simulink model "gm_CornerDetection"  (R2019b)
settings: Solver=FixedStepDiscrete  StartTime=0.0  StopTime=Ts_240p*5  RelTol=1e-3
InitFcn:
  | Ts = 1e-3;
  | Ts_240p = 402*324*Ts;
  | Ts_480p = 525*800*Ts;
undefined symbols (not defined in the file or in its folder): fspecial, gray, Rec, SDTV
libraries: hdlsllib x8, visionhdlfilter x5, visionhdlio x2, simulink x1, visionhdlutilities x1, visionhdlconversions x1, dspvision x1
settings Model: ModifiedByFormat=The MathWorks Inc.  Creator=The MathWorks, Inc.  LastModifiedBy=The MathWorks Inc.
settings DataIOCC: LimitDataPoints=on  SaveFormat=Array  SaveOutput=off  SaveTime=off  ReturnWorkspaceOutputs=off
settings OptimizationCC: BlockReduction=off  ConditionallyExecuteInputs=off  DefaultParameterBehavior=Inlined  LifeSpan=inf
settings DebuggingCC: AlgebraicLoopMsg=error  SolverPrmCheckMsg=warning  InheritedTsInSrcMsg=none  SingleTaskRateTransMsg=error  ParameterPrecisionLossMsg=none  AllowSymbolicDim=off  SFUnexpectedBacktrackingDiag=warning  SFNoUnconditionalDefaultTransitionDiag=warning  SFExecutionAtInitializationDiag=none  IntegerSaturationMsg=none  ArithmeticOperatorsInVariantConditions=warning
settings HardwareCC: ProdBitPerPointer=32  ProdBitPerSizeT=32  ProdBitPerPtrDiffT=32  ProdLargestAtomicFloat=None  ProdIntDivRoundTo=Undefined  ProdEndianess=Unspecified  ProdWordSize=32  ProdHWDeviceType=ASIC/FPGA->ASIC/FPGA  ProdEqTarget=off
settings ModelReferenceCC: PropagateSignalLabelsOutOfModel=off
settings SFSimCC: SimUseLocalCustomCode=off  CustomCodeUndefinedFunction=UseInterfaceOnly
settings RTWCC: RTWUseLocalCustomCode=off
settings CodeAppCC: StateflowObjectComments=on
settings GRTTargetCC: TargetLangStandard=C89/C90 (ANSI)  GeneratePreprocessorConditionals=Disable all
settings ConfigComp: CovMetricSettings=dw  CovHtmlReporting=on  CovSaveCumulativeToWorkspaceVar=on  CovSaveSingleToWorkspaceVar=on  CovShowResultsExplorer=off  CovExternalEMLEnable=off  CovSFcnEnable=off

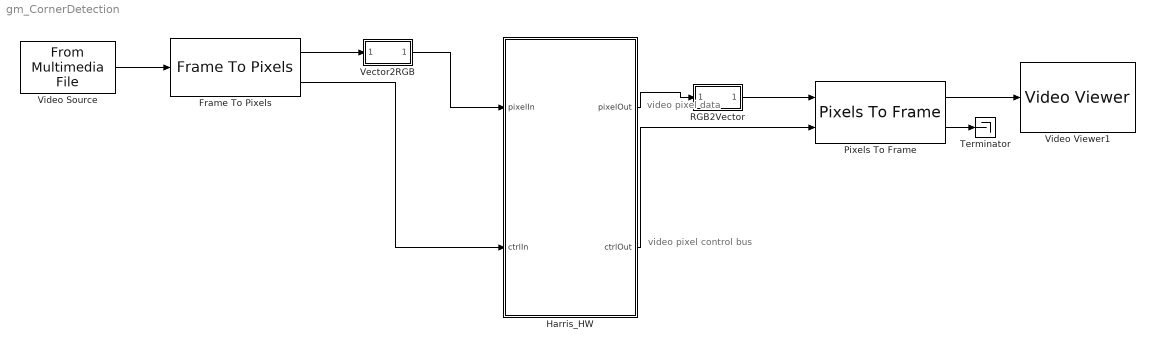
== system gm_CornerDetection ==
  note: video pixel control bus
  note: video pixel data
  Frame To Pixels : visionhdlio/Frame To Pixels  NumComponents=3  NumPixels=1  VideoFormat=480p  ActivePixelsPerLine=32  ActiveVideoLines=18  TotalPixelsPerLine=42  TotalVideoLines=28  StartingActiveLine=6  FrontPorch=5  SampleTime=0
      settings: SourceProductName=Vision HDL Toolbox  SourceProductBaseCode=VT
  Harris_HW : Subsystem  TreatAsAtomicUnit=on
  Pixels To Frame : visionhdlio/Pixels To Frame  NumComponents=3  NumPixels=1  VideoFormat=480p  ActivePixelsPerLine=32  ActiveVideoLines=18  TotalPixelsPerLine=42  TotalVideoLines=28
      settings: SourceProductName=Vision HDL Toolbox  SourceProductBaseCode=VT
  RGB2Vector : Subsystem
  Terminator : Terminator
  Vector2RGB : Subsystem
  Video Source : dspvision/From Multimedia File  inputFilename=D:\RnD\Current_Projects\Musawwir\Frameworks\HW\Musawwir_HW_Zedboard\Custom_IP_Cores\Matlab\Harris\test.jpg  readRange=[1 Inf]  loop=on  numPlays=inf  outputStreams=Video only  videoDataType=uint8  audioDataType=int16  inheritSampleTime=off  userDefinedSampleTime=Ts_480p  noAudioOutput=off  isIntensityVideo=off  fourcc=RGB  colorVideoFormat=One multidimensional signal  outputEOF=off  dataOrg=Column-major  audioFrameSize=1024  computeAudioFrameSize=off  outSamplingMode=Sample based
      settings: SourceProductName=Computer Vision Toolbox  SourceProductBaseCode=VP
  Video Viewer1 : VideoViewer  colormapValue=gray(256)  FigPos=[430.6 726 588 436]
  wires:
  Harris_HW/2(ctrlOut) -> Pixels To Frame/2
  Frame To Pixels/2 -> Harris_HW/2(ctrlIn)
  RGB2Vector/1(RGBVector) -> Pixels To Frame/1
  Frame To Pixels/1 -> Vector2RGB/1(RGBVector)
  Video Source/1 -> Frame To Pixels/1
  Harris_HW/1(pixelOut) -> RGB2Vector/1(RGB)
  Vector2RGB/1(RGB) -> Harris_HW/1(pixelIn)
  Pixels To Frame/1 -> Video Viewer1/1
  Pixels To Frame/2 -> Terminator/1

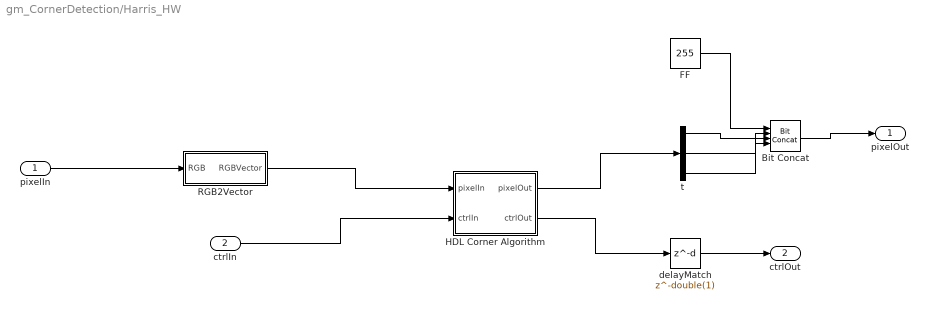
== system gm_CornerDetection/Harris_HW ==
  pixelIn : Inport  OutDataTypeStr=uint32  PortDimensions=1  SampleTime=0.001
  ctrlIn : Inport  Port=2  SampleTime=0.001
  Bit Concat : hdlsllib/Logic and Bit Operations/Bit Concat  numInputs=4
      settings: SourceProductName=Simulink
  FF : Constant  Value=255  OutDataTypeStr=uint8  SampleTime=-1
  HDL Corner Algorithm : Subsystem
  RGB2Vector : Subsystem
  delayMatch : Delay  DelayLength=double(1)  InitialCondition=0  SampleTime=0.001
  t : Demux  Outputs=3
  pixelOut : Outport  VectorParamsAs1DForOutWhenUnconnected=off
  ctrlOut : Outport  Port=2  VectorParamsAs1DForOutWhenUnconnected=off
  wires:
  pixelIn/1 -> RGB2Vector/1(RGB)
  ctrlIn/1 -> HDL Corner Algorithm/2(ctrlIn)
  Bit Concat/1 -> pixelOut/1
  FF/1 -> Bit Concat/1
  HDL Corner Algorithm/1(pixelOut) -> t/1
  delayMatch/1 -> ctrlOut/1
  RGB2Vector/1(RGBVector) -> HDL Corner Algorithm/1(pixelIn)
  t/1 -> Bit Concat/2
  t/2 -> Bit Concat/3
  t/3 -> Bit Concat/4
  HDL Corner Algorithm/2(ctrlOut) -> delayMatch/1

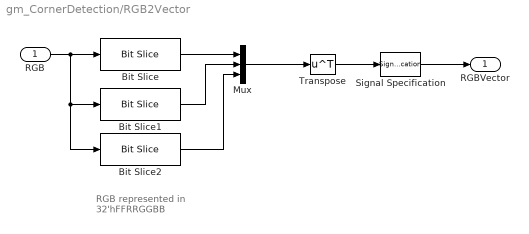
== system gm_CornerDetection/RGB2Vector ==
  note: RGB represented in
      | 32'hFFRRGGBB
  RGB : Inport
  Bit Slice : hdlsllib/Logic and Bit Operations/Bit Slice  lidx=23  ridx=16
  Bit Slice1 : hdlsllib/Logic and Bit Operations/Bit Slice  lidx=15  ridx=8
  Bit Slice2 : hdlsllib/Logic and Bit Operations/Bit Slice  lidx=7  ridx=0
  Mux : Mux  Inputs=3
  Signal Specification : SignalSpecification
  Transpose : Math  Operator=transpose  SaturateOnIntegerOverflow=on
  RGBVector : Outport  VectorParamsAs1DForOutWhenUnconnected=off
  wires:
  Signal Specification/1 -> RGBVector/1
  Transpose/1 -> Signal Specification/1
  RGB/1 -> Bit Slice/1, Bit Slice1/1, Bit Slice2/1
  Bit Slice1/1 -> Mux/2
  Bit Slice2/1 -> Mux/3
  Bit Slice/1 -> Mux/1
  Mux/1 -> Transpose/1

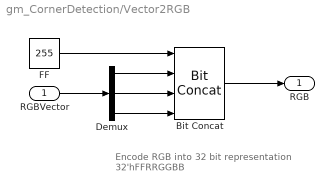
== system gm_CornerDetection/Vector2RGB ==
  note: Encode RGB into 32 bit representation
      | 32'hFFRRGGBB
  RGBVector : Inport
  Bit Concat : hdlsllib/Logic and Bit Operations/Bit Concat  numInputs=4
      settings: SourceProductName=HDL Coder  SourceProductBaseCode=HD
  Demux : Demux  Outputs=3
  FF : Constant  Value=255  OutDataTypeStr=uint8  SampleTime=Ts
  RGB : Outport  VectorParamsAs1DForOutWhenUnconnected=off
  wires:
  Demux/3 -> Bit Concat/4
  Demux/2 -> Bit Concat/3
  Demux/1 -> Bit Concat/2
  FF/1 -> Bit Concat/1
  RGBVector/1 -> Demux/1
  Bit Concat/1 -> RGB/1

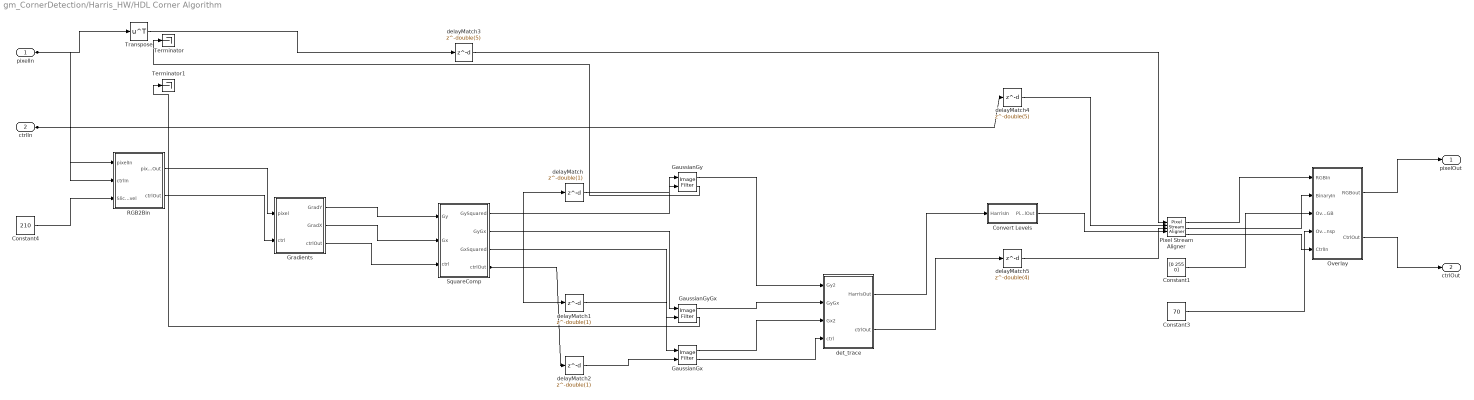
== system gm_CornerDetection/Harris_HW/HDL Corner Algorithm ==
  pixelIn : Inport  OutDataTypeStr=uint8  PortDimensions=[3]  SampleTime=0.001
  ctrlIn : Inport  Port=2  SampleTime=0.001
  Constant1 : Constant  Value=[0 255 0]  VectorParams1D=off  OutDataTypeStr=uint8  SampleTime=-1
  Constant3 : Constant  Value=70  OutDataTypeStr=uint8  SampleTime=-1
  Constant4 : Constant  Value=210  OutDataTypeStr=uint8  SampleTime=-1
  Convert Levels : Subsystem
  GaussianGx : visionhdlfilter/Image Filter  CoefficientsSource=Property  Coefficients=fspecial('gaussian',[5,5],1.5)  PaddingMethod=Constant  PaddingValue=0  LineBufferSize=1024  SimulateUsing=Code generation  roundingMode=Floor  overflowMode=off  CoeffDataTypeStr=fixdt(1,18,21)  CoeffMin=[]  CoeffMax=[]  OutputMin=[]  OutputMax=[]
      settings: SourceProductName=Vision HDL Toolbox  SourceProductBaseCode=VT
  GaussianGy : visionhdlfilter/Image Filter  CoefficientsSource=Property  Coefficients=fspecial('gaussian',[5,5],1.5)  PaddingMethod=Constant  PaddingValue=0  LineBufferSize=1024  SimulateUsing=Code generation  roundingMode=Floor  overflowMode=off  CoeffDataTypeStr=fixdt(1,18,21)  CoeffMin=[]  CoeffMax=[]  OutputMin=[]  OutputMax=[]
      settings: SourceProductName=Vision HDL Toolbox  SourceProductBaseCode=VT
  GaussianGyGx : visionhdlfilter/Image Filter  CoefficientsSource=Property  Coefficients=fspecial('gaussian',[5,5],1.5)  PaddingMethod=Constant  PaddingValue=0  LineBufferSize=1024  SimulateUsing=Code generation  roundingMode=Floor  overflowMode=off  CoeffDataTypeStr=fixdt(1,18,21)  CoeffMin=[]  CoeffMax=[]  OutputMin=[]  OutputMax=[]
      settings: SourceProductName=Vision HDL Toolbox  SourceProductBaseCode=VT
  Gradients : Subsystem
  Overlay : Subsystem
  Pixel Stream Aligner : visionhdlutilities/Pixel Stream Aligner  LineBufferSize=1024  MaximumNumberOfLines=10  SimulateUsing=Code generation
      settings: SourceProductName=Vision HDL Toolbox  SourceProductBaseCode=VT
  RGB2Bin : Subsystem
  SquareComp : Subsystem
  Terminator : Terminator
  Terminator1 : Terminator
  Transpose : Math  Operator=transpose  SaturateOnIntegerOverflow=on
  delayMatch : Delay  DelayLength=double(1)  InitialCondition=0  SampleTime=0.001
  delayMatch1 : Delay  DelayLength=double(1)  InitialCondition=0  SampleTime=0.001
  delayMatch2 : Delay  DelayLength=double(1)  InitialCondition=0  SampleTime=0.001
  delayMatch3 : Delay  DelayLength=double(5)  InitialCondition=0  SampleTime=0.001
  delayMatch4 : Delay  DelayLength=double(5)  InitialCondition=0  SampleTime=0.001
  delayMatch5 : Delay  DelayLength=double(4)  InitialCondition=0  SampleTime=0.001
  det_trace : Subsystem
  pixelOut : Outport  VectorParamsAs1DForOutWhenUnconnected=off
  ctrlOut : Outport  Port=2  VectorParamsAs1DForOutWhenUnconnected=off
  wires:
  delayMatch4/1 -> Pixel Stream Aligner/2
  Constant1/1 -> Overlay/3(OverlayRGB)
  Constant3/1 -> Overlay/4(OverlayTransp)
  Constant4/1 -> RGB2Bin/3(SliceLevel)
  Convert Levels/1(PixelOut) -> Pixel Stream Aligner/3
  GaussianGx/1 -> det_trace/3(Gx2)
  GaussianGx/2 -> det_trace/4(ctrl)
  GaussianGy/1 -> det_trace/1(Gy2)
  GaussianGy/2 -> Terminator/1
  GaussianGyGx/1 -> det_trace/2(GyGx)
  GaussianGyGx/2 -> Terminator1/1
  Gradients/1(GradY) -> SquareComp/1(Gy)
  Gradients/2(GradX) -> SquareComp/2(Gx)
  Gradients/3(ctrlOut) -> SquareComp/3(ctrl)
  Overlay/1(RGBout) -> pixelOut/1
  Overlay/2("CtrlOut ") -> ctrlOut/1
  Pixel Stream Aligner/1 -> Overlay/1(RGBIn)
  Pixel Stream Aligner/2 -> Overlay/2(BinaryIn)
  Pixel Stream Aligner/3 -> Overlay/5(CtrlIn)
  RGB2Bin/1(pixelOut) -> Gradients/1(pixel)
  RGB2Bin/2(ctrlOut) -> Gradients/2(ctrl)
  SquareComp/1(GySquared) -> GaussianGy/1
  SquareComp/2(GyGx) -> GaussianGyGx/1
  SquareComp/3(GxSquared) -> GaussianGx/1
  delayMatch/1 -> GaussianGy/2
  delayMatch3/1 -> Pixel Stream Aligner/1
  det_trace/1(HarrisOut) -> Convert Levels/1(HarrisIn)
  delayMatch5/1 -> Pixel Stream Aligner/4
  pixelIn/1 -> RGB2Bin/1(pixelIn), Transpose/1
  ctrlIn/1 -> delayMatch4/1, RGB2Bin/2(ctrlIn)
  delayMatch1/1 -> GaussianGyGx/2
  delayMatch2/1 -> GaussianGx/2
  SquareComp/4(ctrlOut) -> delayMatch2/1, delayMatch1/1, delayMatch/1
  Transpose/1 -> delayMatch3/1
  det_trace/2(ctrlOut) -> delayMatch5/1

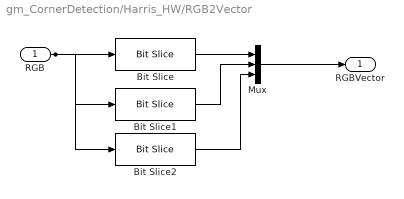
== system gm_CornerDetection/Harris_HW/RGB2Vector ==
  RGB : Inport  OutDataTypeStr=uint32  PortDimensions=1  SampleTime=0.001
  Bit Slice : hdlsllib/Logic and Bit Operations/Bit Slice  lidx=23  ridx=16
  Bit Slice1 : hdlsllib/Logic and Bit Operations/Bit Slice  lidx=15  ridx=8
  Bit Slice2 : hdlsllib/Logic and Bit Operations/Bit Slice  lidx=7  ridx=0
  Mux : Mux  Inputs=3
  RGBVector : Outport  VectorParamsAs1DForOutWhenUnconnected=off
  wires:
  Bit Slice/1 -> Mux/1
  Bit Slice1/1 -> Mux/2
  Bit Slice2/1 -> Mux/3
  Mux/1 -> RGBVector/1
  RGB/1 -> Bit Slice2/1, Bit Slice1/1, Bit Slice/1

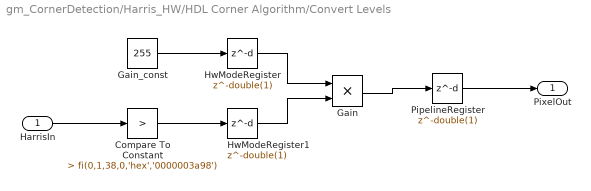
== system gm_CornerDetection/Harris_HW/HDL Corner Algorithm/Convert Levels ==
  HarrisIn : Inport  OutDataTypeStr=fixdt(1, 38, 0)  PortDimensions=1  SampleTime=0.001
  Compare To Constant : simulink/Logic and Bit Operations/Compare To Constant  relop=>  const=fi(0,1,38,0,'hex','0000003a98')  OutDataTypeStr=uint8
  Gain : Product  Inputs=**  OutDataTypeStr=uint8  SampleTime=0.001
  Gain_const : Constant  Value=255  OutDataTypeStr=uint8  SampleTime=-1
  HwModeRegister : Delay  DelayLength=double(1)  InitialCondition=0  SampleTime=0.001
  HwModeRegister1 : Delay  DelayLength=double(1)  InitialCondition=0  SampleTime=0.001
  PipelineRegister : Delay  DelayLength=double(1)  InitialCondition=0  SampleTime=0.001
  PixelOut : Outport  VectorParamsAs1DForOutWhenUnconnected=off
  wires:
  Compare To Constant/1 -> HwModeRegister1/1
  PipelineRegister/1 -> PixelOut/1
  Gain_const/1 -> HwModeRegister/1
  HarrisIn/1 -> Compare To Constant/1
  Gain/1 -> PipelineRegister/1
  HwModeRegister/1 -> Gain/1
  HwModeRegister1/1 -> Gain/2

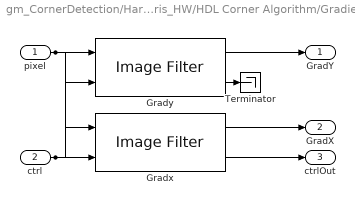
== system gm_CornerDetection/Harris_HW/HDL Corner Algorithm/Gradients ==
  pixel : Inport  OutDataTypeStr=uint8  PortDimensions=1  SampleTime=0.001
  ctrl : Inport  Port=2  SampleTime=0.001
  Gradx : visionhdlfilter/Image Filter  CoefficientsSource=Property  Coefficients=[0,0,0;1, 0,-1;0,0,0]  PaddingMethod=Replicate  PaddingValue=0  LineBufferSize=1024  SimulateUsing=Code generation  roundingMode=Floor  overflowMode=off  CoeffDataTypeStr=fixdt(1,2,0)  CoeffMin=[]  CoeffMax=[]  OutputDataTypeStr=fixdt(1,9,0)  OutputMin=[]  OutputMax=[]
      settings: SourceProductName=Vision HDL Toolbox  SourceProductBaseCode=VT
  Grady : visionhdlfilter/Image Filter  CoefficientsSource=Property  Coefficients=[0,1,0; 0,0,0; 0,-1,0]  PaddingMethod=Replicate  PaddingValue=0  LineBufferSize=1024  SimulateUsing=Code generation  roundingMode=Floor  overflowMode=off  CoeffDataTypeStr=fixdt(1,2,0)  CoeffMin=[]  CoeffMax=[]  OutputDataTypeStr=fixdt(1,9,0)  OutputMin=[]  OutputMax=[]
      settings: SourceProductName=Vision HDL Toolbox  SourceProductBaseCode=VT
  Terminator : Terminator
  GradY : Outport  VectorParamsAs1DForOutWhenUnconnected=off
  GradX : Outport  Port=2  VectorParamsAs1DForOutWhenUnconnected=off
  ctrlOut : Outport  Port=3  VectorParamsAs1DForOutWhenUnconnected=off
  wires:
  Gradx/1 -> GradX/1
  Gradx/2 -> ctrlOut/1
  Grady/1 -> GradY/1
  Grady/2 -> Terminator/1
  pixel/1 -> Gradx/1, Grady/1
  ctrl/1 -> Gradx/2, Grady/2

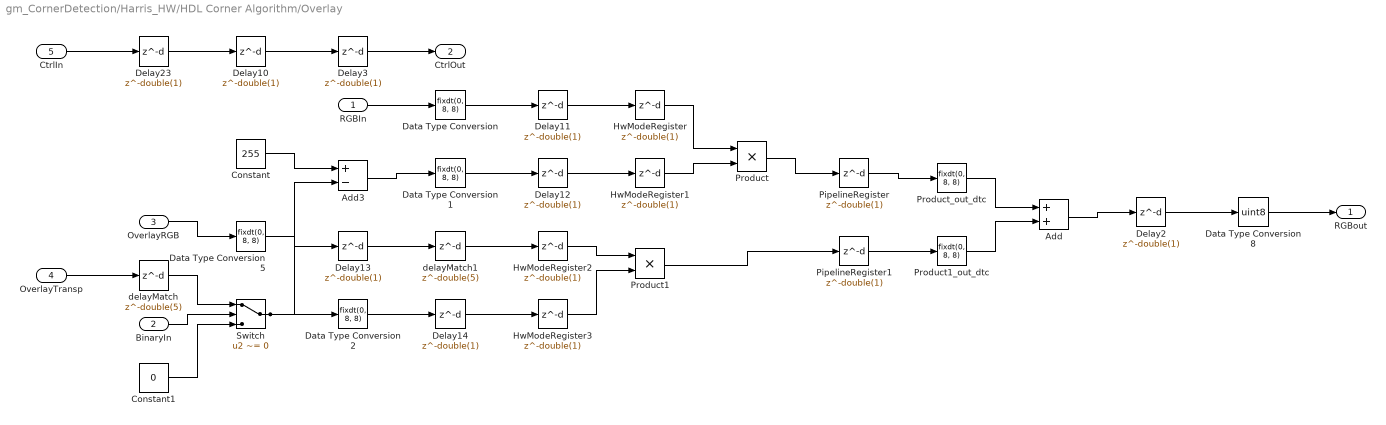
== system gm_CornerDetection/Harris_HW/HDL Corner Algorithm/Overlay ==
  RGBIn : Inport  OutDataTypeStr=uint8  PortDimensions=[1 3]  SampleTime=0.001
  BinaryIn : Inport  Port=2  OutDataTypeStr=uint8  PortDimensions=1  SampleTime=0.001
  OverlayRGB : Inport  Port=3  OutDataTypeStr=uint8  PortDimensions=[1 3]  SampleTime=0.001
  OverlayTransp : Inport  Port=4  OutDataTypeStr=uint8  PortDimensions=1  SampleTime=0.001
  CtrlIn : Inport  Port=5  SampleTime=0.001
  Add : Sum  AccumDataTypeStr=fixdt(0, 9, 8)  OutDataTypeStr=fixdt(0, 8, 8)  SampleTime=0.001
  Add3 : Sum  Inputs=+-  AccumDataTypeStr=uint8  OutDataTypeStr=uint8  SampleTime=0.001
  Constant : Constant  Value=255  OutDataTypeStr=uint8  SampleTime=-1
  Constant1 : Constant  Value=0  OutDataTypeStr=uint8  SampleTime=-1
  Data Type Conversion{,1..2,5} (4 alike) : DataTypeConversion  OutDataTypeStr=fixdt(0, 8, 8)  ConvertRealWorld=Stored Integer (SI)  SampleTime=0.001
  Data Type Conversion8 : DataTypeConversion  OutDataTypeStr=uint8  ConvertRealWorld=Stored Integer (SI)  SampleTime=0.001
  Delay10 : Delay  DelayLength=double(1)  SampleTime=0.001
  Delay{2,11..14} (5 alike) : Delay  DelayLength=double(1)  InitialCondition=0  SampleTime=0.001
  Delay23 : Delay  DelayLength=double(1)  SampleTime=0.001
  Delay3 : Delay  DelayLength=double(1)  SampleTime=0.001
  HwModeRegister{,1..3} (4 alike) : Delay  DelayLength=double(1)  InitialCondition=0  SampleTime=0.001
  PipelineRegister : Delay  DelayLength=double(1)  InitialCondition=0  SampleTime=0.001
  PipelineRegister1 : Delay  DelayLength=double(1)  InitialCondition=0  SampleTime=0.001
  Product : Product  Inputs=**  OutDataTypeStr=fixdt(0, 16, 16)  SampleTime=0.001
  Product1 : Product  Inputs=**  OutDataTypeStr=fixdt(0, 16, 16)  SampleTime=0.001
  Product1_out_dtc : DataTypeConversion  OutDataTypeStr=fixdt(0, 8, 8)  SampleTime=0.001  SaturateOnIntegerOverflow=on
  Product_out_dtc : DataTypeConversion  OutDataTypeStr=fixdt(0, 8, 8)  SampleTime=0.001  SaturateOnIntegerOverflow=on
  Switch : Switch  Criteria=u2 ~= 0  Threshold=double(0)  OutDataTypeStr=uint8  SampleTime=0.001
  delayMatch : Delay  DelayLength=double(5)  InitialCondition=0  SampleTime=0.001
  delayMatch1 : Delay  DelayLength=double(5)  InitialCondition=0  SampleTime=0.001
  RGBout : Outport  VectorParamsAs1DForOutWhenUnconnected=off
  "CtrlOut " : Outport  Port=2  VectorParamsAs1DForOutWhenUnconnected=off
  wires:
  delayMatch/1 -> Switch/1
  Add/1 -> Delay2/1
  Add3/1 -> Data Type Conversion1/1
  Constant/1 -> Add3/1
  Constant1/1 -> Switch/3
  Data Type Conversion/1 -> Delay11/1
  Data Type Conversion1/1 -> Delay12/1
  Data Type Conversion2/1 -> Delay14/1
  Data Type Conversion5/1 -> Delay13/1
  Data Type Conversion8/1 -> RGBout/1
  Delay10/1 -> Delay3/1
  Delay11/1 -> HwModeRegister/1
  Delay12/1 -> HwModeRegister1/1
  delayMatch1/1 -> HwModeRegister2/1
  Delay14/1 -> HwModeRegister3/1
  Delay2/1 -> Data Type Conversion8/1
  Delay23/1 -> Delay10/1
  Delay3/1 -> "CtrlOut "/1
  Product_out_dtc/1 -> Add/1
  Product1_out_dtc/1 -> Add/2
  Switch/1 -> Data Type Conversion2/1, Add3/2
  PipelineRegister/1 -> Product_out_dtc/1
  PipelineRegister1/1 -> Product1_out_dtc/1
  RGBIn/1 -> Data Type Conversion/1
  BinaryIn/1 -> Switch/2
  OverlayRGB/1 -> Data Type Conversion5/1
  OverlayTransp/1 -> delayMatch/1
  CtrlIn/1 -> Delay23/1
  Delay13/1 -> delayMatch1/1
  Product/1 -> PipelineRegister/1
  HwModeRegister/1 -> Product/1
  HwModeRegister1/1 -> Product/2
  Product1/1 -> PipelineRegister1/1
  HwModeRegister2/1 -> Product1/1
  HwModeRegister3/1 -> Product1/2

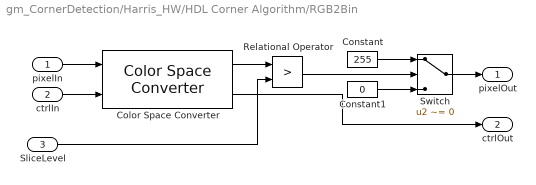
== system gm_CornerDetection/Harris_HW/HDL Corner Algorithm/RGB2Bin ==
  pixelIn : Inport  OutDataTypeStr=uint8  PortDimensions=[3]  SampleTime=0.001
  ctrlIn : Inport  Port=2  SampleTime=0.001
  SliceLevel : Inport  Port=3  OutDataTypeStr=uint8  PortDimensions=1  SampleTime=0.001
  Color Space Converter : visionhdlconversions/Color Space Converter  Conversion=RGB to intensity  ConversionStandard=Rec. 601 (SDTV)  ScanningStandard=1250/50/2:1  SimulateUsing=Code generation
      settings: SourceProductName=Vision HDL Toolbox  SourceProductBaseCode=VT
  Constant : Constant  Value=255  OutDataTypeStr=uint8  SampleTime=-1
  Constant1 : Constant  Value=0  OutDataTypeStr=uint8  SampleTime=-1
  Relational Operator : RelationalOperator  Operator=>  OutDataTypeStr=boolean  RndMeth=Nearest
  Switch : Switch  Criteria=u2 ~= 0
  pixelOut : Outport  VectorParamsAs1DForOutWhenUnconnected=off
  ctrlOut : Outport  Port=2  VectorParamsAs1DForOutWhenUnconnected=off
  wires:
  Color Space Converter/1 -> Relational Operator/1
  Color Space Converter/2 -> ctrlOut/1
  Constant/1 -> Switch/1
  Constant1/1 -> Switch/3
  Relational Operator/1 -> Switch/2
  Switch/1 -> pixelOut/1
  pixelIn/1 -> Color Space Converter/1
  ctrlIn/1 -> Color Space Converter/2
  SliceLevel/1 -> Relational Operator/2

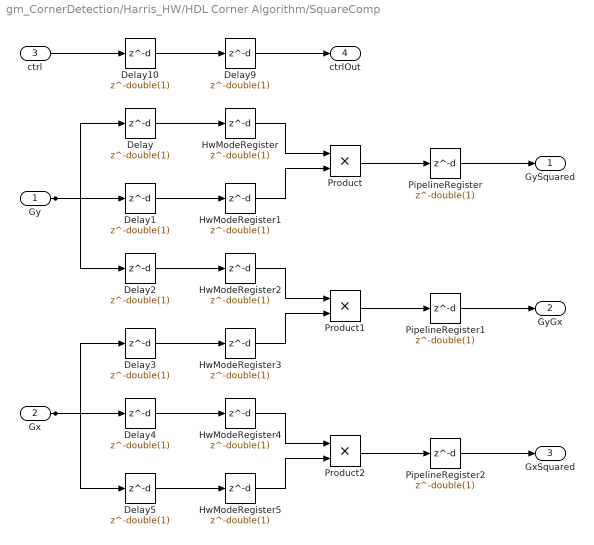
== system gm_CornerDetection/Harris_HW/HDL Corner Algorithm/SquareComp ==
  Gy : Inport  OutDataTypeStr=fixdt(1, 9, 0)  PortDimensions=1  SampleTime=0.001
  Gx : Inport  Port=2  OutDataTypeStr=fixdt(1, 9, 0)  PortDimensions=1  SampleTime=0.001
  ctrl : Inport  Port=3  SampleTime=0.001
  Delay{,1..5} (6 alike) : Delay  DelayLength=double(1)  InitialCondition=0  SampleTime=0.001
  Delay10 : Delay  DelayLength=double(1)  SampleTime=0.001
  Delay9 : Delay  DelayLength=double(1)  SampleTime=0.001
  HwModeRegister{,1..5} (6 alike) : Delay  DelayLength=double(1)  InitialCondition=0  SampleTime=0.001
  PipelineRegister : Delay  DelayLength=double(1)  InitialCondition=0  SampleTime=0.001
  PipelineRegister1 : Delay  DelayLength=double(1)  InitialCondition=0  SampleTime=0.001
  PipelineRegister2 : Delay  DelayLength=double(1)  InitialCondition=0  SampleTime=0.001
  Product : Product  Inputs=**  OutDataTypeStr=fixdt(1, 18, 0)  SampleTime=0.001
  Product1 : Product  Inputs=**  OutDataTypeStr=fixdt(1, 18, 0)  SampleTime=0.001
  Product2 : Product  Inputs=**  OutDataTypeStr=fixdt(1, 18, 0)  SampleTime=0.001
  GySquared : Outport  VectorParamsAs1DForOutWhenUnconnected=off
  GyGx : Outport  Port=2  VectorParamsAs1DForOutWhenUnconnected=off
  GxSquared : Outport  Port=3  VectorParamsAs1DForOutWhenUnconnected=off
  ctrlOut : Outport  Port=4  VectorParamsAs1DForOutWhenUnconnected=off
  wires:
  Delay/1 -> HwModeRegister/1
  Delay1/1 -> HwModeRegister1/1
  Delay10/1 -> Delay9/1
  Delay2/1 -> HwModeRegister2/1
  Delay3/1 -> HwModeRegister3/1
  Delay4/1 -> HwModeRegister4/1
  Delay5/1 -> HwModeRegister5/1
  Delay9/1 -> ctrlOut/1
  PipelineRegister/1 -> GySquared/1
  PipelineRegister1/1 -> GyGx/1
  PipelineRegister2/1 -> GxSquared/1
  Gy/1 -> Delay2/1, Delay1/1, Delay/1
  Gx/1 -> Delay5/1, Delay4/1, Delay3/1
  ctrl/1 -> Delay10/1
  Product/1 -> PipelineRegister/1
  HwModeRegister/1 -> Product/1
  HwModeRegister1/1 -> Product/2
  Product1/1 -> PipelineRegister1/1
  HwModeRegister2/1 -> Product1/1
  HwModeRegister3/1 -> Product1/2
  Product2/1 -> PipelineRegister2/1
  HwModeRegister4/1 -> Product2/1
  HwModeRegister5/1 -> Product2/2

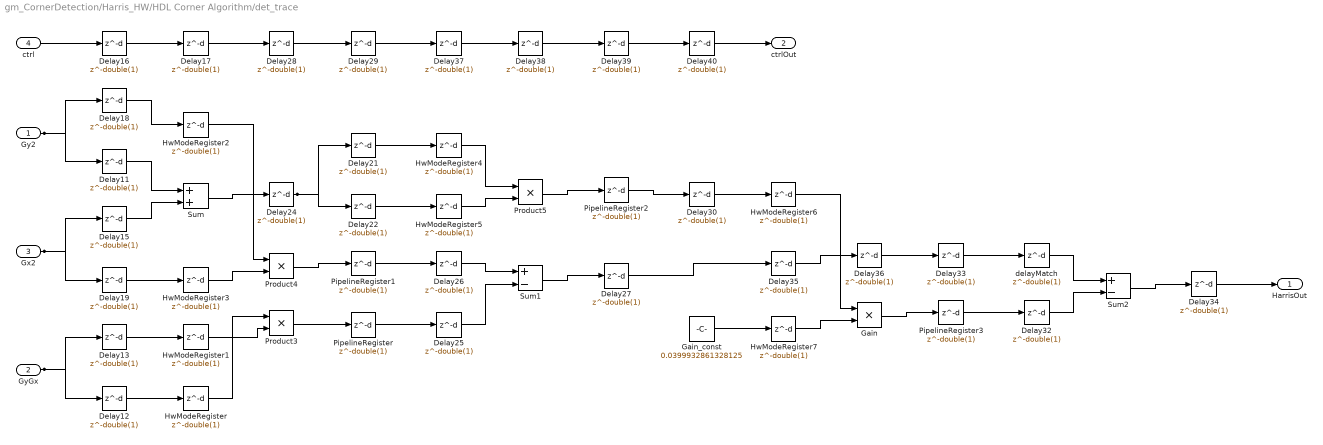
== system gm_CornerDetection/Harris_HW/HDL Corner Algorithm/det_trace ==
  Gy2 : Inport  OutDataTypeStr=fixdt(1, 18, 0)  PortDimensions=1  SampleTime=0.001
  GyGx : Inport  Port=2  OutDataTypeStr=fixdt(1, 18, 0)  PortDimensions=1  SampleTime=0.001
  Gx2 : Inport  Port=3  OutDataTypeStr=fixdt(1, 18, 0)  PortDimensions=1  SampleTime=0.001
  ctrl : Inport  Port=4  SampleTime=0.001
  Delay{11..13,15,18..19,21..22,24..27,30,32..36} (18 alike) : Delay  DelayLength=double(1)  InitialCondition=0  SampleTime=0.001
  Delay{16..17,28..29,37..40} (8 alike) : Delay  DelayLength=double(1)  SampleTime=0.001
  Gain : Product  Inputs=**  OutDataTypeStr=fixdt(1, 36, 0)  SampleTime=0.001
  Gain_const : Constant  Value=0.0399932861328125  OutDataTypeStr=fixdt(0, 16, 16)  SampleTime=-1
  HwModeRegister{,1..7} (8 alike) : Delay  DelayLength=double(1)  InitialCondition=0  SampleTime=0.001
  PipelineRegister{,1..3} (4 alike) : Delay  DelayLength=double(1)  InitialCondition=0  SampleTime=0.001
  Product3 : Product  Inputs=**  OutDataTypeStr=fixdt(1, 36, 0)  SampleTime=0.001
  Product4 : Product  Inputs=**  OutDataTypeStr=fixdt(1, 36, 0)  SampleTime=0.001
  Product5 : Product  Inputs=**  OutDataTypeStr=fixdt(1, 36, 0)  SampleTime=0.001
  Sum : Sum  AccumDataTypeStr=fixdt(1, 19, 0)  OutDataTypeStr=fixdt(1, 18, 0)  SampleTime=0.001
  Sum1 : Sum  Inputs=+-  AccumDataTypeStr=fixdt(1, 37, 0)  OutDataTypeStr=fixdt(1, 37, 0)  SampleTime=0.001
  Sum2 : Sum  Inputs=+-  AccumDataTypeStr=fixdt(1, 38, 0)  OutDataTypeStr=fixdt(1, 38, 0)  SampleTime=0.001
  delayMatch : Delay  DelayLength=double(1)  InitialCondition=0  SampleTime=0.001
  HarrisOut : Outport  VectorParamsAs1DForOutWhenUnconnected=off
  ctrlOut : Outport  Port=2  VectorParamsAs1DForOutWhenUnconnected=off
  wires:
  Delay11/1 -> Sum/1
  Delay12/1 -> HwModeRegister/1
  Delay13/1 -> HwModeRegister1/1
  Delay15/1 -> Sum/2
  Delay16/1 -> Delay17/1
  Delay17/1 -> Delay28/1
  Delay18/1 -> HwModeRegister2/1
  Delay19/1 -> HwModeRegister3/1
  Delay21/1 -> HwModeRegister4/1
  Delay22/1 -> HwModeRegister5/1
  Delay24/1 -> Delay22/1, Delay21/1
  Delay25/1 -> Sum1/2
  Delay26/1 -> Sum1/1
  Delay27/1 -> Delay35/1
  Delay28/1 -> Delay29/1
  Delay29/1 -> Delay37/1
  Delay30/1 -> HwModeRegister6/1
  Delay32/1 -> Sum2/2
  delayMatch/1 -> Sum2/1
  Delay34/1 -> HarrisOut/1
  Delay35/1 -> Delay36/1
  Delay36/1 -> Delay33/1
  Delay37/1 -> Delay38/1
  Delay38/1 -> Delay39/1
  Delay39/1 -> Delay40/1
  Delay40/1 -> ctrlOut/1
  PipelineRegister3/1 -> Delay32/1
  PipelineRegister/1 -> Delay25/1
  PipelineRegister1/1 -> Delay26/1
  PipelineRegister2/1 -> Delay30/1
  Sum/1 -> Delay24/1
  Sum1/1 -> Delay27/1
  Sum2/1 -> Delay34/1
  Gain_const/1 -> HwModeRegister7/1
  Gy2/1 -> Delay18/1, Delay11/1
  GyGx/1 -> Delay13/1, Delay12/1
  Gx2/1 -> Delay19/1, Delay15/1
  ctrl/1 -> Delay16/1
  Delay33/1 -> delayMatch/1
  Product3/1 -> PipelineRegister/1
  HwModeRegister/1 -> Product3/1
  HwModeRegister1/1 -> Product3/2
  Product4/1 -> PipelineRegister1/1
  HwModeRegister2/1 -> Product4/1
  HwModeRegister3/1 -> Product4/2
  Product5/1 -> PipelineRegister2/1
  HwModeRegister4/1 -> Product5/1
  HwModeRegister5/1 -> Product5/2
  Gain/1 -> PipelineRegister3/1
  HwModeRegister6/1 -> Gain/1
  HwModeRegister7/1 -> Gain/2
